simulink model "Single_Phase_SAPF_01mar2018"  (R2017a)
settings: Solver=ode45  StartTime=0.0  StopTime=5  RelTol=1e-3  EnableMultiTasking=on
libraries: powerlib x16, powerlib_meascontrol x2, powerlib_extras x1, simulink x1
settings Model: Creator=Niranjan  LastModifiedBy=Dell
settings DataIOCC: LimitDataPoints=on  SaveFormat=Array
settings OptimizationCC: LifeSpan=inf
settings DebuggingCC: SolverPrmCheckMsg=warning  SFUnexpectedBacktrackingDiag=warning  SFNoUnconditionalDefaultTransitionDiag=warning  SFExecutionAtInitializationDiag=none
settings HardwareCC: ProdBitPerPointer=32  ProdBitPerSizeT=32  ProdBitPerPtrDiffT=32  ProdLargestAtomicFloat=None  ProdIntDivRoundTo=Undefined  ProdEndianess=Unspecified  ProdWordSize=32  ProdHWDeviceType=32-bit Generic
settings ModelReferenceCC: PropagateSignalLabelsOutOfModel=off
settings GRTTargetCC: TargetLangStandard=C89/C90 (ANSI)  GeneratePreprocessorConditionals=Disable all
settings ConfigComp: CovMetricSettings=dw  CovHtmlReporting=on  CovSaveCumulativeToWorkspaceVar=on  CovSaveSingleToWorkspaceVar=on  CovExternalEMLEnable=off  CovSFcnEnable=off

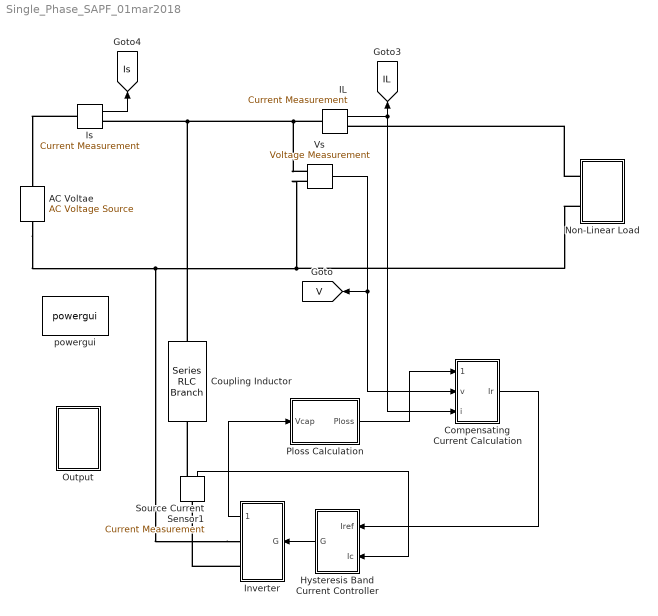
== system Single_Phase_SAPF_01mar2018 ==
  AC Voltae : powerlib/Electrical Sources/AC Voltage Source  Amplitude=311  Phase=0  Frequency=50  SampleTime=0  Measurements=None  BusType=swing  Pref=10e3  Qref=0  Qmin=-inf  Qmax=+inf
  Compensating Current Calculation : Subsystem
  Coupling Inductor : powerlib/Elements/Series RLC Branch  LConnTagsString=__new0  RConnTagsString=__new0  BranchType=RL  Resistance=1  Inductance=0.0035  SetiL0=off  InitialCurrent=0  Capacitance=0.015  Setx0=off  InitialVoltage=0  Measurements=None
  Hysteresis Band Current Controller : Subsystem
  IL : powerlib/Measurements/Current Measurement  PhasorSimulation=off  OutputType=Complex  PSBequivalent=0
  Inverter : Subsystem
  Is : powerlib/Measurements/Current Measurement  PhasorSimulation=off  OutputType=Complex  PSBequivalent=0
  Non-Linear Load : Subsystem
  Output : Subsystem
  Ploss Calculation : Subsystem
  Source Current Sensor1 : powerlib/Measurements/Current Measurement  PhasorSimulation=off  OutputType=Complex  PSBequivalent=0
  Vs : powerlib/Measurements/Voltage Measurement  PhasorSimulation=off  OutputType=Complex  PSBequivalent=0
  powergui : powerlib/powergui  Priority=1  SimulationMode=Discrete  SampleTime=1e-6  frequency=60  Iterations=50  frequencyindice=50  Pbase=100e6  ErrMax=1e-4  UnitsV=kV  UnitsW=MW  buscounter=0  FunctionMessages=off  echomessages=off  EnableUseOfTLC=off  CurrentSourceSwitches=off  DisableSnubberDevices=off  DisableRonSwitches=off  DisableVfSwitches=off  DisplayEquations=off  SolverType=Tustin/Backward Euler (TBE)  Interpol=off  ExternalGateDelay=off  methode=off  Ts=10  x0status=blocks  SPID=off  SwTol=0  HookPort=off  RestoreLinks=warning  ResistiveCurrentMeasurement=off  Frange=[0:2:500]  Ylog=off  Xlog=on  ShowGrid=off  save=off  variable=ZData  structure=0  ZoomFFT=off  StartTime=0.0  cycles=1  DisplayStyle=1  fundamental=60  FreqAxis=off  MaxFrequency=1000  frequencyindicesteady=1  RmsSteady=1  display=off
  tag scope: IL=global, Is=global, V=global
  wires:
  IL/1 -> Compensating Current Calculation/3(i), [IL]
  Vs/1 -> Compensating Current Calculation/2(v), [V]
  Is/1 -> [Is]
  Source Current Sensor1/1 -> Hysteresis Band Current Controller/2(Ic)
  Hysteresis Band Current Controller/1(G) -> Inverter/1(G)
  Inverter/1(Vcap) -> Ploss Calculation/1(Vcap)
  Ploss Calculation/1(Ploss) -> Compensating Current Calculation/1(Ploss)
  Compensating Current Calculation/1(Ir) -> Hysteresis Band Current Controller/1(Iref)
  connections:
  IL/LConn1 -- Vs/LConn1 -- Coupling Inductor/LConn1 -- Is/RConn1
  Inverter/RConn1 -- AC Voltae/LConn1 -- Non-Linear Load/LConn2 -- Vs/LConn2
  Is/LConn1 -- AC Voltae/RConn1
  Inverter/RConn2 -- Source Current Sensor1/LConn1
  Source Current Sensor1/RConn1 -- Coupling Inductor/RConn1
  Non-Linear Load/LConn1 -- IL/RConn1

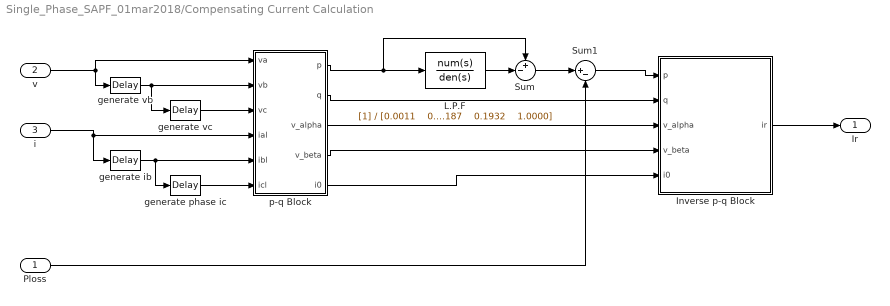
== system Single_Phase_SAPF_01mar2018/Compensating Current Calculation ==
  Ploss : Inport
  v : Inport  Port=2
  i : Inport  Port=3
  Inverse p-q Block : MATLAB Function  TreatAsAtomicUnit=on
  L.P.F : TransferFcn  Denominator="[0.0011    0.0187    0.1932    1.0000]"
  Sum : Sum  Inputs=+-|
  Sum1 : Sum  Inputs=|+-
  generate phase ic : TransportDelay  DelayTime=1/150  BufferSize=10240
  generate ib : TransportDelay  DelayTime=1/150  BufferSize=10240
  generate vb : TransportDelay  DelayTime=1/150  BufferSize=10240
  generate vc : TransportDelay  DelayTime=1/150  BufferSize=10240
  p-q Block : MATLAB Function  TreatAsAtomicUnit=on
  Ir : Outport
  wires:
  p-q Block/1(p) -> Sum/1, L.P.F/1
  Ploss/1 -> Sum1/2
  Sum/1 -> Sum1/1
  Sum1/1 -> Inverse p-q Block/1(p)
  p-q Block/2(q) -> Inverse p-q Block/2(q)
  v/1 -> generate vb/1, p-q Block/1(va)
  i/1 -> generate ib/1, p-q Block/4(ial)
  generate vb/1 -> generate vc/1, p-q Block/2(vb)
  generate vc/1 -> p-q Block/3(vc)
  generate ib/1 -> generate phase ic/1, p-q Block/5(ibl)
  generate phase ic/1 -> p-q Block/6(icl)
  Inverse p-q Block/1(ir) -> Ir/1
  p-q Block/3(v_alpha) -> Inverse p-q Block/3(v_alpha)
  p-q Block/4(v_beta) -> Inverse p-q Block/4(v_beta)
  L.P.F/1 -> Sum/2
  p-q Block/5(i0) -> Inverse p-q Block/5(i0)

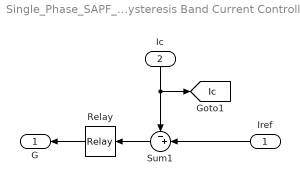
== system Single_Phase_SAPF_01mar2018/Hysteresis Band Current Controller ==
  Iref : Inport
  Ic : Inport  Port=2
  Relay : Relay  OnSwitchValue=0.1  OffSwitchValue=-0.1  ZeroCross=off
  Sum1 : Sum  Inputs=-+|
  G : Outport
  tag scope: Ic=global
  wires:
  Relay/1 -> G/1
  Ic/1 -> Sum1/1, [Ic]
  Sum1/1 -> Relay/1
  Iref/1 -> Sum1/2

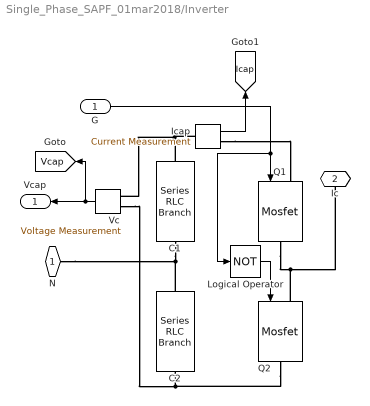
== system Single_Phase_SAPF_01mar2018/Inverter ==
  G : Inport
  C1 : powerlib/Elements/Series RLC Branch  LConnTagsString=__new0  RConnTagsString=__new0  BranchType=C  Resistance=1  Inductance=0.04  SetiL0=off  InitialCurrent=0  Capacitance=500e-6  Setx0=on  InitialVoltage=400  Measurements=None
  C2 : powerlib/Elements/Series RLC Branch  LConnTagsString=__new0  RConnTagsString=__new0  BranchType=C  Resistance=1  Inductance=0.04  SetiL0=off  InitialCurrent=0  Capacitance=500e-6  Setx0=on  InitialVoltage=400  Measurements=None
  Icap : powerlib/Measurements/Current Measurement  PhasorSimulation=off  OutputType=Complex  PSBequivalent=0
  Logical Operator : Logic  Operator=NOT  AllPortsSameDT=off  OutDataTypeStr=boolean
  Q1 : powerlib/Power Electronics/Mosfet  Ron=0.1  Lon=0  Rd=0.01  Vfd=0  IC=0  Rs=1e5  Cs=inf  Measurements=off
  Q2 : powerlib/Power Electronics/Mosfet  Ron=0.1  Lon=0  Rd=0.01  Vfd=0  IC=0  Rs=1e5  Cs=inf  Measurements=off
  Vc : powerlib/Measurements/Voltage Measurement  PhasorSimulation=off  OutputType=Complex  PSBequivalent=0
  N : PMIOPort  Port=1  Side=Right
  Ic : PMIOPort  Port=2  Side=Right
  Vcap : Outport
  tag scope: Icap=global, Vcap=global
  wires:
  Logical Operator/1 -> Q2/1
  G/1 -> Q1/1, Logical Operator/1
  Vc/1 -> [Vcap], Vcap/1
  Icap/1 -> [Icap]
  connections:
  Ic/RConn1 -- Q2/LConn1 -- Q1/RConn1
  Q2/RConn1 -- Vc/LConn2 -- C2/RConn1
  C1/LConn1 -- Icap/LConn1 -- Vc/LConn1
  N/RConn1 -- C2/LConn1 -- C1/RConn1
  Icap/RConn1 -- Q1/LConn1

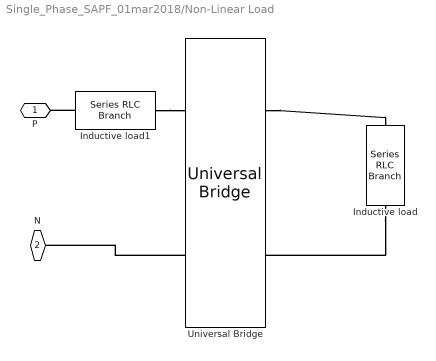
== system Single_Phase_SAPF_01mar2018/Non-Linear Load ==
  Inductive load : powerlib/Elements/Series RLC Branch  LConnTagsString=__new0  RConnTagsString=__new0  BranchType=RL  Resistance=50  Inductance=0.8  SetiL0=off  InitialCurrent=0  Capacitance=0.015  Setx0=off  InitialVoltage=0  Measurements=None
  Inductive load1 : powerlib/Elements/Series RLC Branch  LConnTagsString=__new0  RConnTagsString=__new0  BranchType=L  Resistance=50  Inductance=1e-4  SetiL0=off  InitialCurrent=0  Capacitance=0.015  Setx0=off  InitialVoltage=0  Measurements=None
  Universal Bridge : powerlib/Power Electronics/Universal Bridge  Arms=2  SnubberResistance=1e5  SnubberCapacitance=inf  Device=Diodes  Ron=1e-3  Lon=0  ForwardVoltages="[  0  0  ]"  ForwardVoltage=0  GTOparameters=[ 10e-6 , 20e-6 ]  IGBTparameters=[ 1e-6 , 2e-6 ]  Measurements=None  Measurements_2=None  converterType=Rectifier
  P : PMIOPort  Port=1  Side=Left
  N : PMIOPort  Port=2  Side=Left
  connections:
  Universal Bridge/RConn1 -- Inductive load/LConn1
  Inductive load/RConn1 -- Universal Bridge/RConn2
  Universal Bridge/LConn2 -- N/RConn1
  Inductive load1/LConn1 -- Universal Bridge/LConn1
  Inductive load1/RConn1 -- P/RConn1

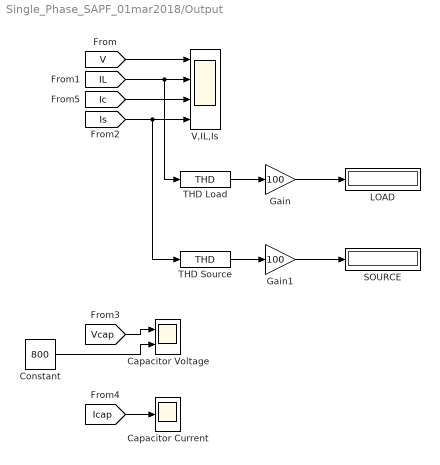
== system Single_Phase_SAPF_01mar2018/Output ==
  Capacitor Current : Scope
  Capacitor Voltage : Scope  NumInputPorts=2
  Constant : Constant  Value=800
  Gain : Gain  Gain=100
  Gain1 : Gain  Gain=100
  LOAD : Display
  SOURCE : Display
  THD Load : powerlib_meascontrol/Measurements/THD  Freq=50  Ts=0
  THD Source : powerlib_meascontrol/Measurements/THD  Freq=50  Ts=0
  V,IL,Is : Scope  NumInputPorts=4
  wires:
  [V] -> V,IL,Is/1
  [Vcap] -> Capacitor Voltage/1
  [Icap] -> Capacitor Current/1
  [Ic] -> V,IL,Is/3
  [Is] -> THD Source/1, V,IL,Is/4
  [IL] -> THD Load/1, V,IL,Is/2
  Gain/1 -> LOAD/1
  Gain1/1 -> SOURCE/1
  THD Load/1 -> Gain/1
  THD Source/1 -> Gain1/1
  Constant/1 -> Capacitor Voltage/2

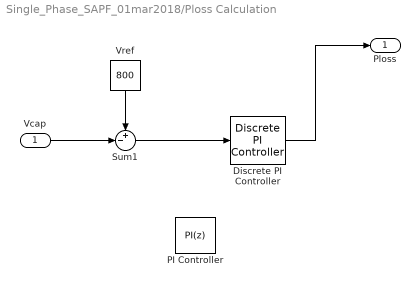
== system Single_Phase_SAPF_01mar2018/Ploss Calculation ==
  Vcap : Inport
  Discrete PI Controller : powerlib_extras/Discrete  Control Blocks/Discrete PI Controller  Kp=1  Ki=0  Par_Limits=[1e6 -1e6]  Init=0  Ts=1e-6
  PI Controller : simulink/Continuous/PID Controller  Controller=PI  TimeDomain=Discrete-time  SampleTime=1e-6  IntegratorMethod=Forward Euler  FilterMethod=Forward Euler  Form=Parallel  UseFilter=on  ControllerParametersSource=internal  P=5  I=1.3  D=0  N=100  InitialConditionSource=internal  InitialConditionForIntegrator=0  InitialConditionForFilter=0  ExternalReset=none  LimitOutput=off  UpperSaturationLimit=inf  LowerSaturationLimit=-inf  LinearizeAsGain=off  AntiWindupMode=none  Kb=1  TrackingMode=off  Kt=1  PParamMin=[]  PParamMax=[]  IParamMin=[]  IParamMax=[]  DParamMin=[]  DParamMax=[]  NParamMin=[]  NParamMax=[]  KbParamMin=[]  KbParamMax=[]  KtParamMin=[]  KtParamMax=[]  POutMin=[]  POutMax=[]  IOutMin=[]  IOutMax=[]  DOutMin=[]  DOutMax=[]  NOutMin=[]  NOutMax=[]  KbOutMin=[]  KbOutMax=[]  KtOutMin=[]  KtOutMax=[]  IntegratorOutMin=[]  IntegratorOutMax=[]  FilterOutMin=[]  FilterOutMax=[]  SumOutMin=[]  SumOutMax=[]  SumI1OutMin=[]  SumI1OutMax=[]  SumI2OutMin=[]  SumI2OutMax=[]  SumI3OutMin=[]  SumI3OutMax=[]  SumDOutMin=[]  SumDOutMax=[]  SaturationOutMin=[]  SaturationOutMax=[]  IntegratorContinuousStateAttributes=''  IntegratorStateMustResolveToSignalObject=off  IntegratorRTWStateStorageClass=Auto  FilterContinuousStateAttributes=''  FilterStateMustResolveToSignalObject=off  FilterRTWStateStorageClass=Auto  DifferentiatorICPrevScaledInput=0  DifferentiatorOutMin=[]  DifferentiatorOutMax=[]  InitialConditionSetting=State (most efficient)
  Sum1 : Sum  Inputs=+-|
  Vref : Constant  Value=800
  Ploss : Outport
  wires:
  Vref/1 -> Sum1/1
  Vcap/1 -> Sum1/2
  Sum1/1 -> Discrete PI Controller/1
  Discrete PI Controller/1 -> Ploss/1

== matlab function Single_Phase_SAPF_01mar2018/Compensating Current Calculation/Inverse p-q Block ==
  data: p input; q input; v_alpha input; v_beta input; ir output; i0 input
function ir = fcn(p,q,v_alpha,v_beta,i0)
%#codegen
i_alpha=(v_alpha.*p+v_beta.*q)/(v_alpha.^2+v_beta.^2);
i_beta=(v_beta.*p-v_alpha.*q)/(v_alpha.^2+v_beta.^2);
ir=sqrt(2/3)*(i0/sqrt(2)+i_alpha);

== matlab function Single_Phase_SAPF_01mar2018/Compensating Current Calculation/p-q Block ==
  data: va input; p output; vb input; vc input; ial input; ibl input; icl input; q output; v_alpha output; v_beta output; i0 output
function [p,q,v_alpha,v_beta,i0]= fcn(va,vb,vc,ial,ibl,icl)
%#codegen
v_alpha=(va-vb/2-vc/2)*sqrt(2/3);
v_beta=(vb-vc)/sqrt(2);
i0=(ial+ibl+icl)/sqrt(3);
il_alpha=(ial-ibl/2-icl/2)*sqrt(2/3);
il_beta=(ibl-icl)/sqrt(2);
p=v_alpha.*il_alpha+v_beta.*il_beta;
q=v_beta.*il_alpha-v_alpha.*il_beta;
